simulink model "Facies"  (R2024a)
settings: Solver=VariableStepAuto  StartTime=0.0  StopTime=6  RelTol=1e-3
(part 2 of 2)

== matlab function Facies/media ==
  data: u input; y output
function y = media(u)

y = mean(u);

== matlab function Facies/media2 ==
  data: u input; y output
function y = media(u)

y = mean(u);

== matlab function Facies/media3 ==
  data: u input; y output
function y = media(u)

y = mean(u);

== matlab function Facies/media1 ==
  data: u input; y output
function y = media(u)

y = mean(u);
